simulink model "mZC"  (R2021b)
settings: Solver=VariableStepAuto  StartTime=0.0  StopTime=10.0  RelTol=1e-3
settings Model: Creator=anitschk  LastModifiedBy=anitschk

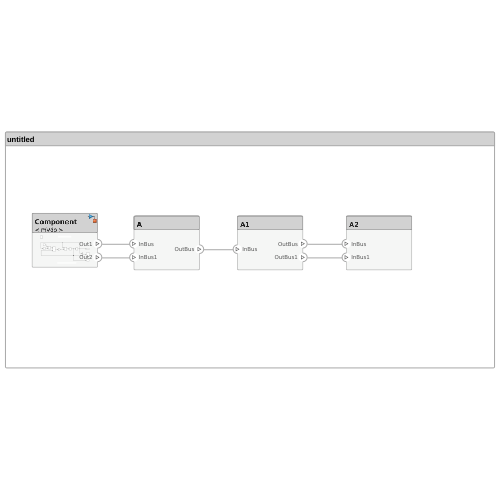
[thumbnail: Simulink's stored preview of the top-level diagram]
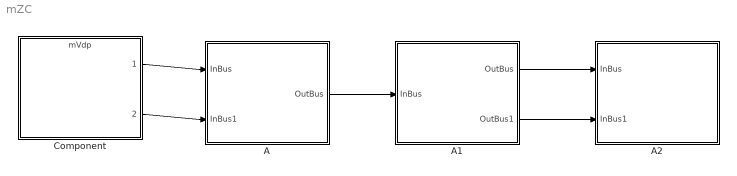
== system mZC ==
  A : Subsystem
      settings: PortSchema="{\"entries\":[{\"content\":{\"headerSize\":26,\"margin\":15,\"minimumSpacing\":25,\"sides\":[{\"content\":{\"connectorIds\":[\"In1\",\"In2\"]},\"type\":\"ConnectorPlacement.EquallySpacedRectSide\",\"uuid\":\"47eadd57-f61a-46ab-8544-95fc6583d676\"},{\"content\":{\"connectorIds\":[\"Out1\"],\"side\":\"RIGHT\"},\"type\":\"ConnectorPlacement.EquallySpacedRectSide\",\"uuid\":\"fe63b160-fd0f-4914-9524-7eebf5a6f2dc\"},{\"content\":{\"connectorIds\":[],\"side\":\"TOP\"},\"type\":\"ConnectorPlacement.EquallySpacedRectSide\",\"uuid\":\"bc52174a-bb25-4aeb-94b7-20602e66f067\"}]},\"type\":\"ConnectorPlacement.EquallySpacedConnector\",\"uuid\":\"31530ed4-202b-4fbf-850e-efda93d090c9\"}],\"packageUris\":[\"http://schema.mathworks.com/mf0/Connector/R2020b\"],\"version\":\"1.0\"}"
  A1 : Subsystem
      settings: PortSchema="{\"entries\":[{\"content\":{\"headerSize\":26,\"margin\":15,\"minimumSpacing\":25,\"sides\":[{\"content\":{\"connectorIds\":[\"In1\"]},\"type\":\"ConnectorPlacement.EquallySpacedRectSide\",\"uuid\":\"47eadd57-f61a-46ab-8544-95fc6583d676\"},{\"content\":{\"connectorIds\":[\"Out1\",\"Out2\"],\"side\":\"RIGHT\"},\"type\":\"ConnectorPlacement.EquallySpacedRectSide\",\"uuid\":\"fe63b160-fd0f-4914-9524-7eebf5a6f2dc\"},{\"content\":{\"connectorIds\":[],\"side\":\"TOP\"},\"type\":\"ConnectorPlacement.EquallySpacedRectSide\",\"uuid\":\"bc52174a-bb25-4aeb-94b7-20602e66f067\"}]},\"type\":\"ConnectorPlacement.EquallySpacedConnector\",\"uuid\":\"31530ed4-202b-4fbf-850e-efda93d090c9\"}],\"packageUris\":[\"http://schema.mathworks.com/mf0/Connector/R2020b\"],\"version\":\"1.0\"}"
  A2 : Subsystem
      settings: PortSchema="{\"entries\":[{\"content\":{\"headerSize\":26,\"margin\":15,\"minimumSpacing\":25,\"sides\":[{\"content\":{\"connectorIds\":[\"In1\",\"In2\"]},\"type\":\"ConnectorPlacement.EquallySpacedRectSide\",\"uuid\":\"47eadd57-f61a-46ab-8544-95fc6583d676\"},{\"content\":{\"connectorIds\":[],\"side\":\"RIGHT\"},\"type\":\"ConnectorPlacement.EquallySpacedRectSide\",\"uuid\":\"fe63b160-fd0f-4914-9524-7eebf5a6f2dc\"},{\"content\":{\"connectorIds\":[],\"side\":\"TOP\"},\"type\":\"ConnectorPlacement.EquallySpacedRectSide\",\"uuid\":\"bc52174a-bb25-4aeb-94b7-20602e66f067\"}]},\"type\":\"ConnectorPlacement.EquallySpacedConnector\",\"uuid\":\"31530ed4-202b-4fbf-850e-efda93d090c9\"}],\"packageUris\":[\"http://schema.mathworks.com/mf0/Connector/R2020b\"],\"version\":\"1.0\"}"
  Component : ModelReference  ModelNameDialog=mVdp  SimulationMode=Normal  ModelReferenceVersion=4.0
      settings: PortSchema="{\"entries\":[{\"content\":{\"headerSize\":38,\"margin\":15,\"minimumSpacing\":25,\"sides\":[{\"content\":{\"connectorIds\":[]},\"type\":\"ConnectorPlacement.EquallySpacedRectSide\",\"uuid\":\"3eedf7c3-f8d3-4763-bec4-b7ec770b4e71\"},{\"content\":{\"connectorIds\":[\"Out1\",\"Out2\"],\"side\":\"RIGHT\"},\"type\":\"ConnectorPlacement.EquallySpacedRectSide\",\"uuid\":\"b9adaaed-715c-46eb-941b-09c2ba984293\"},{\"content\":{\"connectorIds\":[],\"side\":\"TOP\"},\"type\":\"ConnectorPlacement.EquallySpacedRectSide\",\"uuid\":\"d06ce2ec-33e3-449d-9408-c04356a9b14f\"}]},\"type\":\"ConnectorPlacement.EquallySpacedConnector\",\"uuid\":\"3ce1f0aa-781e-43b8-a6cf-b2f7862f196e\"}],\"packageUris\":[\"http://schema.mathworks.com/mf0/Connector/R2020b\"],\"version\":\"1.0\"}"
  wires:
  A/1(OutBus) -> A1/1(InBus)
  A1/1(OutBus) -> A2/1(InBus)
  A1/2(OutBus1) -> A2/2(InBus1)
  Component/1 -> A/1(InBus)
  Component/2 -> A/2(InBus1)

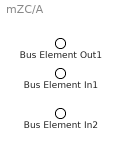
== system mZC/A ==
  Bus Element In1 : Inport  PortName=InBus
  Bus Element In2 : Inport  Port=2  PortName=InBus1
  Bus Element Out1 : Outport  PortName=OutBus

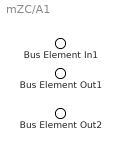
== system mZC/A1 ==
  Bus Element In1 : Inport  PortName=InBus
  Bus Element Out1 : Outport  PortName=OutBus
  Bus Element Out2 : Outport  Port=2  PortName=OutBus1

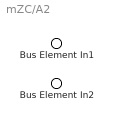
== system mZC/A2 ==
  Bus Element In1 : Inport  PortName=InBus
  Bus Element In2 : Inport  Port=2  PortName=InBus1
